simulink model "line_choices_snt"  (R2025b)
settings: Solver=ode45  StartTime=0.0  StopTime=10.0  RelTol=1e-3  EnableMultiTasking=on
values from neighbouring files (symbols this model uses):
  ft2km = 0.0003048    [IEEE_123_data.m]    (also in IEEE_123_data_fault.m)
undefined symbols (not defined in the file or in its folder): C_1, find_system, L_1, R_1
libraries: fl_lib x156, nesl_utility x24
(part 1 of 2)
settings Model: Creator=gdudgeon  LastModifiedBy=gdudgeon
settings SolverCC: AlgebraicLoopSolver=TrustRegion
settings DataIOCC: LimitDataPoints=on  SaveFormat=Array  ReturnWorkspaceOutputs=off
settings OptimizationCC: ExpressionDepthLimit=2147483647.0  LifeSpan=inf
settings DebuggingCC: UnderspecifiedInitializationDetection=Classic  MergeDetectMultiDrivingBlocksExec=none  SolverPrmCheckMsg=warning  UnconnectedInputMsg=warning  UnconnectedOutputMsg=warning  UnconnectedLineMsg=warning  StateNameClashWarn=warning  SFUnexpectedBacktrackingDiag=warning  SFNoUnconditionalDefaultTransitionDiag=warning  SFExecutionAtInitializationDiag=none  ArithmeticOperatorsInVariantConditions=warning
settings HardwareCC: ProdBitPerPointer=32.0  ProdBitPerSizeT=32.0  ProdBitPerPtrDiffT=32.0  ProdLargestAtomicFloat=None  ProdIntDivRoundTo=Undefined  ProdEndianess=Unspecified  ProdWordSize=32.0  ProdHWDeviceType=32-bit Generic
settings ModelReferenceCC: EnableRefExpFcnMdlSchedulingChecks=on  PropagateSignalLabelsOutOfModel=off
settings SFSimCC: SimUseLocalCustomCode=off  CustomCodeUndefinedFunction=UseInterfaceOnly
settings RTWCC: RTWUseLocalCustomCode=off  GPUComputeCapability=3.5
settings CodeAppCC: StateflowObjectComments=on
settings GRTTargetCC: TargetLangStandard=C89/C90 (ANSI)
settings ConfigComp: CovMetricSettings=dw  CovSaveCumulativeToWorkspaceVar=on  CovSaveSingleToWorkspaceVar=on  CovExternalEMLEnable=off  CovSFcnEnable=off
settings SimscapeCC: SimscapeNormalizeSystem=off

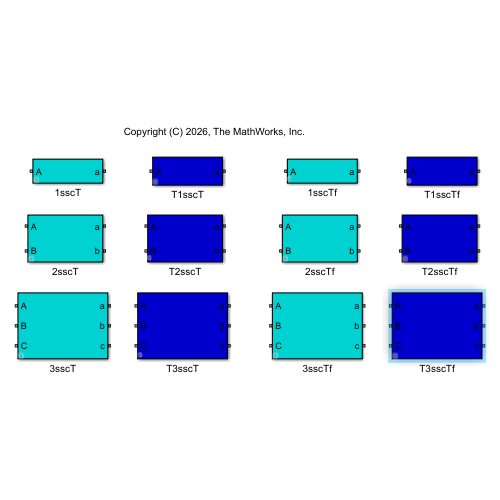
[thumbnail: Simulink's stored preview of the top-level diagram]
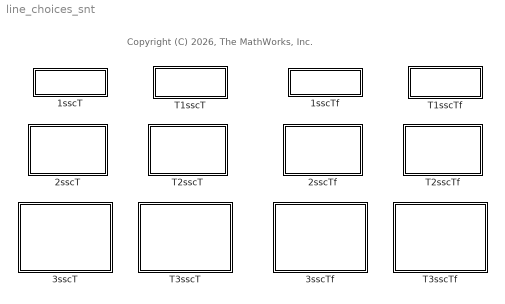
== system line_choices_snt ==
  note: Copyright (C) 2026, The MathWorks, Inc.
  1sscT : Subsystem  mask{from_bus=1, to_bus=7, config=1, length=300}
      mask prompts: from_bus "From Bus"; to_bus "To Bus"; config "Configuration"; length "Length (ft)"
  1sscTf : Subsystem  mask{from_bus=1, to_bus=7, config=1, length=300}
      mask prompts: from_bus "From Bus"; to_bus "To Bus"; config "Configuration"; length "Length (ft)"
  2sscT : Subsystem  mask{from_bus=1, to_bus=7, config=1, length=300}
      mask prompts: from_bus "From Bus"; to_bus "To Bus"; config "Configuration"; length "Length (ft)"
  2sscTf : Subsystem  mask{from_bus=1, to_bus=7, config=1, length=300}
      mask prompts: from_bus "From Bus"; to_bus "To Bus"; config "Configuration"; length "Length (ft)"
  3sscT : Subsystem  mask{from_bus=1, to_bus=7, config=1, length=300}
      mask prompts: from_bus "From Bus"; to_bus "To Bus"; config "Configuration"; length "Length (ft)"
  3sscTf : Subsystem  mask{from_bus=1, to_bus=7, config=1, length=300}
      mask prompts: from_bus "From Bus"; to_bus "To Bus"; config "Configuration"; length "Length (ft)"
  T1sscT : Subsystem  mask{from_bus=67, to_bus=160, config=6, length=350}
      mask prompts: from_bus "From Bus"; to_bus "To Bus"; config "Configuration"; length "Length (ft)"
  T1sscTf : Subsystem  mask{from_bus=67, to_bus=160, config=6, length=350}
      mask prompts: from_bus "From Bus"; to_bus "To Bus"; config "Configuration"; length "Length (ft)"
  T2sscT : Subsystem  mask{from_bus=67, to_bus=160, config=6, length=350}
      mask prompts: from_bus "From Bus"; to_bus "To Bus"; config "Configuration"; length "Length (ft)"
  T2sscTf : Subsystem  mask{from_bus=67, to_bus=160, config=6, length=350}
      mask prompts: from_bus "From Bus"; to_bus "To Bus"; config "Configuration"; length "Length (ft)"
  T3sscT : Subsystem  mask{from_bus=67, to_bus=160, config=6, length=350}
      mask prompts: from_bus "From Bus"; to_bus "To Bus"; config "Configuration"; length "Length (ft)"
  T3sscTf : Subsystem  mask{from_bus=67, to_bus=160, config=6, length=350}
      mask prompts: from_bus "From Bus"; to_bus "To Bus"; config "Configuration"; length "Length (ft)"

== system line_choices_snt/1sscT ==
  Pi-Section Line : Subsystem  mask{Resistance=R_1, Inductance=L_1, Capacitance=C_1, Length=300*ft2km}
      mask prompts: Resistance "R (3x3) ohms/km"; Inductance "L (3x3) H/km"; Capacitance "C (3x3) F/km"; Length "length (km)"
      mask init:
      | R = Resistance*Length;
      | L = Inductance*Length;
      | C = Capacitance*Length;
  A : PMIOPort  Side=Left
  a : PMIOPort  Port=2  Side=Right
  tag scope: Iabc_1=global
  wires:
  Pi-Section Line/1(Imeas) -> [Iabc_1]
  connections:
  a/RConn1 -- Pi-Section Line/RConn1
  A/RConn1 -- Pi-Section Line/LConn1

== system line_choices_snt/1sscTf ==
  Pi-Section Line : Subsystem  mask{Resistance=R_1, Inductance=L_1, Capacitance=C_1, Length=300*ft2km}
      mask prompts: Resistance "R (3x3) ohms/km"; Inductance "L (3x3) H/km"; Capacitance "C (3x3) F/km"; Length "length (km)"
      mask init:
      | R = Resistance*Length;
      | L = Inductance*Length;
      | C = Capacitance*Length;
  A : PMIOPort  Side=Left
  a : PMIOPort  Port=2  Side=Right
  tag scope: Iabc_1=global
  wires:
  Pi-Section Line/1(Imeas) -> [Iabc_1]
  connections:
  A/RConn1 -- Pi-Section Line/LConn1
  a/RConn1 -- Pi-Section Line/RConn1

== system line_choices_snt/2sscT ==
  Pi-Section Line : Subsystem  mask{Resistance=R_1, Inductance=L_1, Capacitance=C_1, Length=300*ft2km}
      mask prompts: Resistance "R (3x3) ohms/km"; Inductance "L (3x3) H/km"; Capacitance "C (3x3) F/km"; Length "length (km)"
      mask init:
      | R = Resistance*Length;
      | L = Inductance*Length;
      | C = Capacitance*Length;
  A : PMIOPort  Side=Left
  a : PMIOPort  Port=2  Side=Right
  B : PMIOPort  Port=3  Side=Left
  b : PMIOPort  Port=4  Side=Right
  tag scope: Iabc_1=global
  wires:
  Pi-Section Line/1(Imeas) -> [Iabc_1]
  connections:
  a/RConn1 -- Pi-Section Line/RConn1
  b/RConn1 -- Pi-Section Line/RConn2
  A/RConn1 -- Pi-Section Line/LConn1
  B/RConn1 -- Pi-Section Line/LConn2

== system line_choices_snt/2sscTf ==
  Pi-Section Line : Subsystem  mask{Resistance=R_1, Inductance=L_1, Capacitance=C_1, Length=300*ft2km}
      mask prompts: Resistance "R (3x3) ohms/km"; Inductance "L (3x3) H/km"; Capacitance "C (3x3) F/km"; Length "length (km)"
      mask init:
      | R = Resistance*Length;
      | L = Inductance*Length;
      | C = Capacitance*Length;
  A : PMIOPort  Side=Left
  a : PMIOPort  Port=2  Side=Right
  B : PMIOPort  Port=3  Side=Left
  b : PMIOPort  Port=4  Side=Right
  tag scope: Iabc_1=global
  wires:
  Pi-Section Line/1(Imeas) -> [Iabc_1]
  connections:
  B/RConn1 -- Pi-Section Line/LConn2
  A/RConn1 -- Pi-Section Line/LConn1
  b/RConn1 -- Pi-Section Line/RConn2
  a/RConn1 -- Pi-Section Line/RConn1

== system line_choices_snt/3sscT ==
  Pi-Section Line : Subsystem  mask{Resistance=R_1, Inductance=L_1, Capacitance=C_1/2, Length=300*ft2km}
      mask prompts: Resistance "R (3x3) ohms/km"; Inductance "L (3x3) H/km"; Capacitance "C (3x3) F/km"; Length "length (km)"
      mask init:
      | R = Resistance*Length;
      | L = Inductance*Length;
      | C = Capacitance*Length;
  A : PMIOPort  Side=Left
  a : PMIOPort  Port=2  Side=Right
  B : PMIOPort  Port=3  Side=Left
  b : PMIOPort  Port=4  Side=Right
  C : PMIOPort  Port=5  Side=Left
  c : PMIOPort  Port=6  Side=Right
  tag scope: Iabc_1=global
  wires:
  Pi-Section Line/1(Imeas) -> [Iabc_1]
  connections:
  c/RConn1 -- Pi-Section Line/RConn3
  b/RConn1 -- Pi-Section Line/RConn2
  a/RConn1 -- Pi-Section Line/RConn1
  C/RConn1 -- Pi-Section Line/LConn3
  B/RConn1 -- Pi-Section Line/LConn2
  A/RConn1 -- Pi-Section Line/LConn1

== system line_choices_snt/3sscTf ==
  Pi-Section Line : Subsystem  mask{Resistance=R_1, Inductance=L_1, Capacitance=C_1/2, Length=300*ft2km}
      mask prompts: Resistance "R (3x3) ohms/km"; Inductance "L (3x3) H/km"; Capacitance "C (3x3) F/km"; Length "length (km)"
      mask init:
      | R = Resistance*Length;
      | L = Inductance*Length;
      | C = Capacitance*Length;
  A : PMIOPort  Side=Left
  a : PMIOPort  Port=2  Side=Right
  B : PMIOPort  Port=3  Side=Left
  b : PMIOPort  Port=4  Side=Right
  C : PMIOPort  Port=5  Side=Left
  c : PMIOPort  Port=6  Side=Right
  tag scope: Iabc_1=global
  wires:
  Pi-Section Line/1(Imeas) -> [Iabc_1]
  connections:
  A/RConn1 -- Pi-Section Line/LConn1
  B/RConn1 -- Pi-Section Line/LConn2
  C/RConn1 -- Pi-Section Line/LConn3
  a/RConn1 -- Pi-Section Line/RConn1
  b/RConn1 -- Pi-Section Line/RConn2
  c/RConn1 -- Pi-Section Line/RConn3

== system line_choices_snt/T1sscT ==
  OLTC : Subsystem  LoadFcn=find_system(gcs,'FollowLinks', 'on', 'LookUnderMasks', 'all');
  Pi-Section Line : Subsystem  mask{Resistance=R_1, Inductance=L_1, Capacitance=C_1, Length=300*ft2km}
      mask prompts: Resistance "R (3x3) ohms/km"; Inductance "L (3x3) H/km"; Capacitance "C (3x3) F/km"; Length "length (km)"
      mask init:
      | R = Resistance*Length;
      | L = Inductance*Length;
      | C = Capacitance*Length;
  A : PMIOPort  Side=Left
  a : PMIOPort  Port=2  Side=Right
  tag scope: Iabc_1=global
  wires:
  Pi-Section Line/1(Imeas) -> [Iabc_1]
  connections:
  A/RConn1 -- OLTC/LConn1
  Pi-Section Line/RConn1 -- a/RConn1
  Pi-Section Line/LConn1 -- OLTC/RConn1

== system line_choices_snt/T1sscTf ==
  OLTC : Subsystem  LoadFcn=find_system(gcs,'FollowLinks', 'on', 'LookUnderMasks', 'all');
  Pi-Section Line : Subsystem  mask{Resistance=R_1, Inductance=L_1, Capacitance=C_1, Length=300*ft2km}
      mask prompts: Resistance "R (3x3) ohms/km"; Inductance "L (3x3) H/km"; Capacitance "C (3x3) F/km"; Length "length (km)"
      mask init:
      | R = Resistance*Length;
      | L = Inductance*Length;
      | C = Capacitance*Length;
  A : PMIOPort  Side=Left
  a : PMIOPort  Port=2  Side=Right
  tag scope: Iabc_1=global
  wires:
  Pi-Section Line/1(Imeas) -> [Iabc_1]
  connections:
  Pi-Section Line/LConn1 -- OLTC/RConn1
  Pi-Section Line/RConn1 -- a/RConn1
  A/RConn1 -- OLTC/LConn1

== system line_choices_snt/T2sscT ==
  OLTC : Subsystem  LoadFcn=find_system(gcs,'FollowLinks', 'on', 'LookUnderMasks', 'all');
  Pi-Section Line : Subsystem  mask{Resistance=R_1, Inductance=L_1, Capacitance=C_1, Length=300*ft2km}
      mask prompts: Resistance "R (3x3) ohms/km"; Inductance "L (3x3) H/km"; Capacitance "C (3x3) F/km"; Length "length (km)"
      mask init:
      | R = Resistance*Length;
      | L = Inductance*Length;
      | C = Capacitance*Length;
  A : PMIOPort  Side=Left
  a : PMIOPort  Port=2  Side=Right
  B : PMIOPort  Port=3  Side=Left
  b : PMIOPort  Port=4  Side=Right
  tag scope: Iabc_1=global
  wires:
  Pi-Section Line/1(Imeas) -> [Iabc_1]
  connections:
  a/RConn1 -- Pi-Section Line/RConn1
  b/RConn1 -- Pi-Section Line/RConn2
  A/RConn1 -- OLTC/LConn1
  B/RConn1 -- OLTC/LConn2
  Pi-Section Line/LConn2 -- OLTC/RConn2
  Pi-Section Line/LConn1 -- OLTC/RConn1

== system line_choices_snt/T2sscTf ==
  OLTC : Subsystem  LoadFcn=find_system(gcs,'FollowLinks', 'on', 'LookUnderMasks', 'all');
  Pi-Section Line : Subsystem  mask{Resistance=R_1, Inductance=L_1, Capacitance=C_1, Length=300*ft2km}
      mask prompts: Resistance "R (3x3) ohms/km"; Inductance "L (3x3) H/km"; Capacitance "C (3x3) F/km"; Length "length (km)"
      mask init:
      | R = Resistance*Length;
      | L = Inductance*Length;
      | C = Capacitance*Length;
  A : PMIOPort  Side=Left
  a : PMIOPort  Port=2  Side=Right
  B : PMIOPort  Port=3  Side=Left
  b : PMIOPort  Port=4  Side=Right
  tag scope: Iabc_1=global
  wires:
  Pi-Section Line/1(Imeas) -> [Iabc_1]
  connections:
  Pi-Section Line/LConn1 -- OLTC/RConn1
  Pi-Section Line/LConn2 -- OLTC/RConn2
  B/RConn1 -- OLTC/LConn2
  A/RConn1 -- OLTC/LConn1
  b/RConn1 -- Pi-Section Line/RConn2
  a/RConn1 -- Pi-Section Line/RConn1

== system line_choices_snt/T3sscT ==
  OLTC : Subsystem  LoadFcn=find_system(gcs,'FollowLinks', 'on', 'LookUnderMasks', 'all');
  Pi-Section Line : Subsystem  mask{Resistance=R_1, Inductance=L_1, Capacitance=C_1/2, Length=300*ft2km}
      mask prompts: Resistance "R (3x3) ohms/km"; Inductance "L (3x3) H/km"; Capacitance "C (3x3) F/km"; Length "length (km)"
      mask init:
      | R = Resistance*Length;
      | L = Inductance*Length;
      | C = Capacitance*Length;
  A : PMIOPort  Side=Left
  a : PMIOPort  Port=2  Side=Right
  B : PMIOPort  Port=3  Side=Left
  b : PMIOPort  Port=4  Side=Right
  C : PMIOPort  Port=5  Side=Left
  c : PMIOPort  Port=6  Side=Right
  tag scope: Iabc_1=global
  wires:
  Pi-Section Line/1(Imeas) -> [Iabc_1]
  connections:
  A/RConn1 -- OLTC/LConn1
  B/RConn1 -- OLTC/LConn2
  OLTC/LConn3 -- C/RConn1
  c/RConn1 -- Pi-Section Line/RConn3
  Pi-Section Line/RConn1 -- a/RConn1
  b/RConn1 -- Pi-Section Line/RConn2
  Pi-Section Line/LConn2 -- OLTC/RConn2
  OLTC/RConn1 -- Pi-Section Line/LConn1
  OLTC/RConn3 -- Pi-Section Line/LConn3

== system line_choices_snt/T3sscTf ==
  OLTC : Subsystem  LoadFcn=find_system(gcs,'FollowLinks', 'on', 'LookUnderMasks', 'all');
  Pi-Section Line : Subsystem  mask{Resistance=R_1, Inductance=L_1, Capacitance=C_1/2, Length=300*ft2km}
      mask prompts: Resistance "R (3x3) ohms/km"; Inductance "L (3x3) H/km"; Capacitance "C (3x3) F/km"; Length "length (km)"
      mask init:
      | R = Resistance*Length;
      | L = Inductance*Length;
      | C = Capacitance*Length;
  A : PMIOPort  Side=Left
  a : PMIOPort  Port=2  Side=Right
  B : PMIOPort  Port=3  Side=Left
  b : PMIOPort  Port=4  Side=Right
  C : PMIOPort  Port=5  Side=Left
  c : PMIOPort  Port=6  Side=Right
  tag scope: Iabc_1=global
  wires:
  Pi-Section Line/1(Imeas) -> [Iabc_1]
  connections:
  OLTC/RConn3 -- Pi-Section Line/LConn3
  OLTC/RConn1 -- Pi-Section Line/LConn1
  Pi-Section Line/LConn2 -- OLTC/RConn2
  b/RConn1 -- Pi-Section Line/RConn2
  Pi-Section Line/RConn1 -- a/RConn1
  c/RConn1 -- Pi-Section Line/RConn3
  OLTC/LConn3 -- C/RConn1
  B/RConn1 -- OLTC/LConn2
  A/RConn1 -- OLTC/LConn1

== system line_choices_snt/1sscT/Pi-Section Line ==
  Electrical Reference : fl_lib/Electrical/Electrical Elements/Electrical Reference
  Electrical Reference1 : fl_lib/Electrical/Electrical Elements/Electrical Reference
  Mutual C1 : SimscapeComponentBlock  SourceFile=multi_coupled_C  ComponentPath=multi_coupled_C  ComponentVariants="[\"multi_coupled_C\"]"  ComponentVariantNames="[\"multi_coupled_C\"]"  ClassName=multi_coupled_C  SchemaVersion=1  noph=1  C=C F
      settings: CopyFcn=simscape.sscblock.internal.componentBlockCallback(gcbh,'COPY')  PreCopyFcn=simscape.sscblock.internal.componentBlockCallback(gcbh,'PRECOPY')  PreDeleteFcn=simscape.sscblock.internal.componentBlockCallback(gcbh,'PREDELETE')  InternalSimscapePortConfiguration="{\"Bottom\":[],\"Left\":[{\"id\":\"p\",\"label\":\"p\",\"type\":\"foundation.electrical.electrical\"}],\"Right\":[{\"id\":\"n\",\"label\":\"n\",\"type\":\"foundation.electrical.electrical\"}],\"Top\":[]}"
      mask Type: Multi-Phase Coupled C
  Mutual C2 : SimscapeComponentBlock  SourceFile=multi_coupled_C  ComponentPath=multi_coupled_C  ComponentVariants="[\"multi_coupled_C\"]"  ComponentVariantNames="[\"multi_coupled_C\"]"  ClassName=multi_coupled_C  SchemaVersion=1  noph=1  C=C F
      settings: CopyFcn=simscape.sscblock.internal.componentBlockCallback(gcbh,'COPY')  PreCopyFcn=simscape.sscblock.internal.componentBlockCallback(gcbh,'PRECOPY')  PreDeleteFcn=simscape.sscblock.internal.componentBlockCallback(gcbh,'PREDELETE')  InternalSimscapePortConfiguration="{\"Bottom\":[],\"Left\":[{\"id\":\"p\",\"label\":\"p\",\"type\":\"foundation.electrical.electrical\"}],\"Right\":[{\"id\":\"n\",\"label\":\"n\",\"type\":\"foundation.electrical.electrical\"}],\"Top\":[]}"
      mask Type: Multi-Phase Coupled C
  Mutual RL : SimscapeComponentBlock  SourceFile=multi_coupled_RL  ComponentPath=multi_coupled_RL  ComponentVariants="[\"multi_coupled_RL\"]"  ComponentVariantNames="[\"multi_coupled_RL\"]"  ClassName=multi_coupled_RL  SchemaVersion=1  noph=1  R=R Ohm  L=L H
      settings: CopyFcn=simscape.sscblock.internal.componentBlockCallback(gcbh,'COPY')  PreCopyFcn=simscape.sscblock.internal.componentBlockCallback(gcbh,'PRECOPY')  PreDeleteFcn=simscape.sscblock.internal.componentBlockCallback(gcbh,'PREDELETE')  InternalSimscapePortConfiguration="{\"Bottom\":[],\"Left\":[{\"id\":\"p\",\"label\":\"p\",\"type\":\"foundation.electrical.electrical\"}],\"Right\":[{\"id\":\"n\",\"label\":\"n\",\"type\":\"foundation.electrical.electrical\"}],\"Top\":[]}"
      mask Type: Multi-Phase Coupled RL
  PS-Simulink Converter : nesl_utility/PS-Simulink Converter  PhysicalDomain=network_engine_domain  SubClassName=ps_output  LeftPortType=input  RightPortType=output  PseudoPeriodic=off  Frequencies=[]  VectorFormat=inherit  Unit=inherit  AffineConversion=off
  Simscape Component : SimscapeComponentBlock  SourceFile=multi_current  ComponentPath=multi_current  ComponentVariants="[\"multi_current\"]"  ComponentVariantNames="[\"multi_current\"]"  ClassName=multi_current  SchemaVersion=1  noph=1
      settings: CopyFcn=simscape.sscblock.internal.componentBlockCallback(gcbh,'COPY')  PreCopyFcn=simscape.sscblock.internal.componentBlockCallback(gcbh,'PRECOPY')  PreDeleteFcn=simscape.sscblock.internal.componentBlockCallback(gcbh,'PREDELETE')  InternalSimscapePortConfiguration="{\"Bottom\":[],\"Left\":[{\"id\":\"p\",\"label\":\"+\",\"type\":\"foundation.electrical.electrical\"}],\"Right\":[{\"id\":\"I\",\"label\":\"I\",\"type\":\"output\"},{\"id\":\"n\",\"label\":\"-\",\"type\":\"foundation.electrical.electrical\"}],\"Top\":[]}"
      mask Type: Multi-Phase Current Sensor
  A : PMIOPort  Side=Left
  a : PMIOPort  Port=2  Side=Right
  Imeas : Outport
  wires:
  PS-Simulink Converter/1 -> Imeas/1
  connections:
  Mutual RL/LConn1 -- Simscape Component/RConn2 -- Mutual C1/LConn1
  Mutual RL/RConn1 -- a/RConn1 -- Mutual C2/LConn1
  Mutual C1/RConn1 -- Electrical Reference/LConn1
  Mutual C2/RConn1 -- Electrical Reference1/LConn1
  Simscape Component/LConn1 -- A/RConn1
  PS-Simulink Converter/LConn1 -- Simscape Component/RConn1

== system line_choices_snt/1sscTf/Pi-Section Line ==
  Electrical Reference : fl_lib/Electrical/Electrical Elements/Electrical Reference
  Electrical Reference1 : fl_lib/Electrical/Electrical Elements/Electrical Reference
  Mutual C1 : SimscapeComponentBlock  SourceFile=multi_coupled_C  ComponentPath=multi_coupled_C  ComponentVariants="[\"multi_coupled_C\"]"  ComponentVariantNames="[\"multi_coupled_C\"]"  ClassName=multi_coupled_C  SchemaVersion=1  noph=1  C=C F
      settings: CopyFcn=simscape.sscblock.internal.componentBlockCallback(gcbh,'COPY')  PreCopyFcn=simscape.sscblock.internal.componentBlockCallback(gcbh,'PRECOPY')  PreDeleteFcn=simscape.sscblock.internal.componentBlockCallback(gcbh,'PREDELETE')  InternalSimscapePortConfiguration="{\"Bottom\":[],\"Left\":[{\"id\":\"p\",\"label\":\"p\",\"type\":\"foundation.electrical.electrical\"}],\"Right\":[{\"id\":\"n\",\"label\":\"n\",\"type\":\"foundation.electrical.electrical\"}],\"Top\":[]}"
      mask Type: Multi-Phase Coupled C
  Mutual C2 : SimscapeComponentBlock  SourceFile=multi_coupled_C  ComponentPath=multi_coupled_C  ComponentVariants="[\"multi_coupled_C\"]"  ComponentVariantNames="[\"multi_coupled_C\"]"  ClassName=multi_coupled_C  SchemaVersion=1  noph=1  C=C F
      settings: CopyFcn=simscape.sscblock.internal.componentBlockCallback(gcbh,'COPY')  PreCopyFcn=simscape.sscblock.internal.componentBlockCallback(gcbh,'PRECOPY')  PreDeleteFcn=simscape.sscblock.internal.componentBlockCallback(gcbh,'PREDELETE')  InternalSimscapePortConfiguration="{\"Bottom\":[],\"Left\":[{\"id\":\"p\",\"label\":\"p\",\"type\":\"foundation.electrical.electrical\"}],\"Right\":[{\"id\":\"n\",\"label\":\"n\",\"type\":\"foundation.electrical.electrical\"}],\"Top\":[]}"
      mask Type: Multi-Phase Coupled C
  Mutual RL : SimscapeComponentBlock  SourceFile=multi_coupled_RL  ComponentPath=multi_coupled_RL  ComponentVariants="[\"multi_coupled_RL\"]"  ComponentVariantNames="[\"multi_coupled_RL\"]"  ClassName=multi_coupled_RL  SchemaVersion=1  noph=1  R=R Ohm  L=L H
      settings: CopyFcn=simscape.sscblock.internal.componentBlockCallback(gcbh,'COPY')  PreCopyFcn=simscape.sscblock.internal.componentBlockCallback(gcbh,'PRECOPY')  PreDeleteFcn=simscape.sscblock.internal.componentBlockCallback(gcbh,'PREDELETE')  InternalSimscapePortConfiguration="{\"Bottom\":[],\"Left\":[{\"id\":\"p\",\"label\":\"p\",\"type\":\"foundation.electrical.electrical\"}],\"Right\":[{\"id\":\"n\",\"label\":\"n\",\"type\":\"foundation.electrical.electrical\"}],\"Top\":[]}"
      mask Type: Multi-Phase Coupled RL
  PS-Simulink Converter : nesl_utility/PS-Simulink Converter  PhysicalDomain=network_engine_domain  SubClassName=ps_output  LeftPortType=input  RightPortType=output  PseudoPeriodic=off  Frequencies=[]  VectorFormat=inherit  Unit=inherit  AffineConversion=off
  Simscape Component : SimscapeComponentBlock  SourceFile=multi_current  ComponentPath=multi_current  ComponentVariants="[\"multi_current\"]"  ComponentVariantNames="[\"multi_current\"]"  ClassName=multi_current  SchemaVersion=1  noph=1
      settings: CopyFcn=simscape.sscblock.internal.componentBlockCallback(gcbh,'COPY')  PreCopyFcn=simscape.sscblock.internal.componentBlockCallback(gcbh,'PRECOPY')  PreDeleteFcn=simscape.sscblock.internal.componentBlockCallback(gcbh,'PREDELETE')  InternalSimscapePortConfiguration="{\"Bottom\":[],\"Left\":[{\"id\":\"p\",\"label\":\"+\",\"type\":\"foundation.electrical.electrical\"}],\"Right\":[{\"id\":\"I\",\"label\":\"I\",\"type\":\"output\"},{\"id\":\"n\",\"label\":\"-\",\"type\":\"foundation.electrical.electrical\"}],\"Top\":[]}"
      mask Type: Multi-Phase Current Sensor
  A : PMIOPort  Side=Left
  a : PMIOPort  Port=2  Side=Right
  Imeas : Outport
  wires:
  PS-Simulink Converter/1 -> Imeas/1
  connections:
  PS-Simulink Converter/LConn1 -- Simscape Component/RConn1
  Simscape Component/LConn1 -- A/RConn1
  Mutual C2/RConn1 -- Electrical Reference1/LConn1
  Mutual C1/RConn1 -- Electrical Reference/LConn1
  Mutual C2/LConn1 -- a/RConn1 -- Mutual RL/RConn1
  Mutual C1/LConn1 -- Simscape Component/RConn2 -- Mutual RL/LConn1

== system line_choices_snt/2sscT/Pi-Section Line ==
  Array Connection{,1..3} (4 alike) : SimscapeArrayConnection
  Electrical Reference : fl_lib/Electrical/Electrical Elements/Electrical Reference
  Electrical Reference1 : fl_lib/Electrical/Electrical Elements/Electrical Reference
  Mutual C1 : SimscapeComponentBlock  SourceFile=multi_coupled_C  ComponentPath=multi_coupled_C  ComponentVariants="[\"multi_coupled_C\"]"  ComponentVariantNames="[\"multi_coupled_C\"]"  ClassName=multi_coupled_C  SchemaVersion=1  noph=2  C=C F
      settings: CopyFcn=simscape.sscblock.internal.componentBlockCallback(gcbh,'COPY')  PreCopyFcn=simscape.sscblock.internal.componentBlockCallback(gcbh,'PRECOPY')  PreDeleteFcn=simscape.sscblock.internal.componentBlockCallback(gcbh,'PREDELETE')  InternalSimscapePortConfiguration="{\"Bottom\":[],\"Left\":[{\"id\":\"p\",\"label\":\"p\",\"type\":\"foundation.electrical.electrical\"}],\"Right\":[{\"id\":\"n\",\"label\":\"n\",\"type\":\"foundation.electrical.electrical\"}],\"Top\":[]}"
      mask Type: Multi-Phase Coupled C
  Mutual C2 : SimscapeComponentBlock  SourceFile=multi_coupled_C  ComponentPath=multi_coupled_C  ComponentVariants="[\"multi_coupled_C\"]"  ComponentVariantNames="[\"multi_coupled_C\"]"  ClassName=multi_coupled_C  SchemaVersion=1  noph=2  C=C F
      settings: CopyFcn=simscape.sscblock.internal.componentBlockCallback(gcbh,'COPY')  PreCopyFcn=simscape.sscblock.internal.componentBlockCallback(gcbh,'PRECOPY')  PreDeleteFcn=simscape.sscblock.internal.componentBlockCallback(gcbh,'PREDELETE')  InternalSimscapePortConfiguration="{\"Bottom\":[],\"Left\":[{\"id\":\"p\",\"label\":\"p\",\"type\":\"foundation.electrical.electrical\"}],\"Right\":[{\"id\":\"n\",\"label\":\"n\",\"type\":\"foundation.electrical.electrical\"}],\"Top\":[]}"
      mask Type: Multi-Phase Coupled C
  Mutual RL : SimscapeComponentBlock  SourceFile=multi_coupled_RL  ComponentPath=multi_coupled_RL  ComponentVariants="[\"multi_coupled_RL\"]"  ComponentVariantNames="[\"multi_coupled_RL\"]"  ClassName=multi_coupled_RL  SchemaVersion=1  noph=2  R=R Ohm  L=L H
      settings: CopyFcn=simscape.sscblock.internal.componentBlockCallback(gcbh,'COPY')  PreCopyFcn=simscape.sscblock.internal.componentBlockCallback(gcbh,'PRECOPY')  PreDeleteFcn=simscape.sscblock.internal.componentBlockCallback(gcbh,'PREDELETE')  InternalSimscapePortConfiguration="{\"Bottom\":[],\"Left\":[{\"id\":\"p\",\"label\":\"p\",\"type\":\"foundation.electrical.electrical\"}],\"Right\":[{\"id\":\"n\",\"label\":\"n\",\"type\":\"foundation.electrical.electrical\"}],\"Top\":[]}"
      mask Type: Multi-Phase Coupled RL
  PS-Simulink Converter : nesl_utility/PS-Simulink Converter  PhysicalDomain=network_engine_domain  SubClassName=ps_output  LeftPortType=input  RightPortType=output  PseudoPeriodic=off  Frequencies=[]  VectorFormat=inherit  Unit=inherit  AffineConversion=off
  Simscape Component : SimscapeComponentBlock  SourceFile=multi_current  ComponentPath=multi_current  ComponentVariants="[\"multi_current\"]"  ComponentVariantNames="[\"multi_current\"]"  ClassName=multi_current  SchemaVersion=1  noph=2
      settings: CopyFcn=simscape.sscblock.internal.componentBlockCallback(gcbh,'COPY')  PreCopyFcn=simscape.sscblock.internal.componentBlockCallback(gcbh,'PRECOPY')  PreDeleteFcn=simscape.sscblock.internal.componentBlockCallback(gcbh,'PREDELETE')  InternalSimscapePortConfiguration="{\"Bottom\":[],\"Left\":[{\"id\":\"p\",\"label\":\"+\",\"type\":\"foundation.electrical.electrical\"}],\"Right\":[{\"id\":\"I\",\"label\":\"I\",\"type\":\"output\"},{\"id\":\"n\",\"label\":\"-\",\"type\":\"foundation.electrical.electrical\"}],\"Top\":[]}"
      mask Type: Multi-Phase Current Sensor
  A : PMIOPort  Side=Left
  B : PMIOPort  Port=2  Side=Left
  a : PMIOPort  Port=3  Side=Right
  b : PMIOPort  Port=4  Side=Right
  Imeas : Outport
  wires:
  PS-Simulink Converter/1 -> Imeas/1
  connections:
  Mutual RL/RConn1 -- Array Connection1/RConn1 -- Mutual C2/LConn1
  Mutual C1/LConn1 -- Simscape Component/RConn2 -- Mutual RL/LConn1
  PS-Simulink Converter/LConn1 -- Simscape Component/RConn1
  Array Connection/RConn1 -- Simscape Component/LConn1
  A/RConn1 -- Array Connection/LConn1
  B/RConn1 -- Array Connection/LConn2
  a/RConn1 -- Array Connection1/LConn1
  b/RConn1 -- Array Connection1/LConn2
  Array Connection2/RConn1 -- Mutual C1/RConn1
  Array Connection3/RConn1 -- Mutual C2/RConn1
  Array Connection2/LConn1 -- Electrical Reference/LConn1 -- Array Connection2/LConn2
  Array Connection3/LConn1 -- Electrical Reference1/LConn1 -- Array Connection3/LConn2

== system line_choices_snt/2sscTf/Pi-Section Line ==
  Array Connection{,1..3} (4 alike) : SimscapeArrayConnection
  Electrical Reference : fl_lib/Electrical/Electrical Elements/Electrical Reference
  Electrical Reference1 : fl_lib/Electrical/Electrical Elements/Electrical Reference
  Mutual C1 : SimscapeComponentBlock  SourceFile=multi_coupled_C  ComponentPath=multi_coupled_C  ComponentVariants="[\"multi_coupled_C\"]"  ComponentVariantNames="[\"multi_coupled_C\"]"  ClassName=multi_coupled_C  SchemaVersion=1  noph=2  C=C F
      settings: CopyFcn=simscape.sscblock.internal.componentBlockCallback(gcbh,'COPY')  PreCopyFcn=simscape.sscblock.internal.componentBlockCallback(gcbh,'PRECOPY')  PreDeleteFcn=simscape.sscblock.internal.componentBlockCallback(gcbh,'PREDELETE')  InternalSimscapePortConfiguration="{\"Bottom\":[],\"Left\":[{\"id\":\"p\",\"label\":\"p\",\"type\":\"foundation.electrical.electrical\"}],\"Right\":[{\"id\":\"n\",\"label\":\"n\",\"type\":\"foundation.electrical.electrical\"}],\"Top\":[]}"
      mask Type: Multi-Phase Coupled C
  Mutual C2 : SimscapeComponentBlock  SourceFile=multi_coupled_C  ComponentPath=multi_coupled_C  ComponentVariants="[\"multi_coupled_C\"]"  ComponentVariantNames="[\"multi_coupled_C\"]"  ClassName=multi_coupled_C  SchemaVersion=1  noph=2  C=C F
      settings: CopyFcn=simscape.sscblock.internal.componentBlockCallback(gcbh,'COPY')  PreCopyFcn=simscape.sscblock.internal.componentBlockCallback(gcbh,'PRECOPY')  PreDeleteFcn=simscape.sscblock.internal.componentBlockCallback(gcbh,'PREDELETE')  InternalSimscapePortConfiguration="{\"Bottom\":[],\"Left\":[{\"id\":\"p\",\"label\":\"p\",\"type\":\"foundation.electrical.electrical\"}],\"Right\":[{\"id\":\"n\",\"label\":\"n\",\"type\":\"foundation.electrical.electrical\"}],\"Top\":[]}"
      mask Type: Multi-Phase Coupled C
  Mutual RL : SimscapeComponentBlock  SourceFile=multi_coupled_RL  ComponentPath=multi_coupled_RL  ComponentVariants="[\"multi_coupled_RL\"]"  ComponentVariantNames="[\"multi_coupled_RL\"]"  ClassName=multi_coupled_RL  SchemaVersion=1  noph=2  R=R Ohm  L=L H
      settings: CopyFcn=simscape.sscblock.internal.componentBlockCallback(gcbh,'COPY')  PreCopyFcn=simscape.sscblock.internal.componentBlockCallback(gcbh,'PRECOPY')  PreDeleteFcn=simscape.sscblock.internal.componentBlockCallback(gcbh,'PREDELETE')  InternalSimscapePortConfiguration="{\"Bottom\":[],\"Left\":[{\"id\":\"p\",\"label\":\"p\",\"type\":\"foundation.electrical.electrical\"}],\"Right\":[{\"id\":\"n\",\"label\":\"n\",\"type\":\"foundation.electrical.electrical\"}],\"Top\":[]}"
      mask Type: Multi-Phase Coupled RL
  PS-Simulink Converter : nesl_utility/PS-Simulink Converter  PhysicalDomain=network_engine_domain  SubClassName=ps_output  LeftPortType=input  RightPortType=output  PseudoPeriodic=off  Frequencies=[]  VectorFormat=inherit  Unit=inherit  AffineConversion=off
  Simscape Component : SimscapeComponentBlock  SourceFile=multi_current  ComponentPath=multi_current  ComponentVariants="[\"multi_current\"]"  ComponentVariantNames="[\"multi_current\"]"  ClassName=multi_current  SchemaVersion=1  noph=2
      settings: CopyFcn=simscape.sscblock.internal.componentBlockCallback(gcbh,'COPY')  PreCopyFcn=simscape.sscblock.internal.componentBlockCallback(gcbh,'PRECOPY')  PreDeleteFcn=simscape.sscblock.internal.componentBlockCallback(gcbh,'PREDELETE')  InternalSimscapePortConfiguration="{\"Bottom\":[],\"Left\":[{\"id\":\"p\",\"label\":\"+\",\"type\":\"foundation.electrical.electrical\"}],\"Right\":[{\"id\":\"I\",\"label\":\"I\",\"type\":\"output\"},{\"id\":\"n\",\"label\":\"-\",\"type\":\"foundation.electrical.electrical\"}],\"Top\":[]}"
      mask Type: Multi-Phase Current Sensor
  A : PMIOPort  Side=Left
  B : PMIOPort  Port=2  Side=Left
  a : PMIOPort  Port=3  Side=Right
  b : PMIOPort  Port=4  Side=Right
  Imeas : Outport
  wires:
  PS-Simulink Converter/1 -> Imeas/1
  connections:
  Array Connection3/LConn2 -- Electrical Reference1/LConn1 -- Array Connection3/LConn1
  Array Connection2/LConn2 -- Electrical Reference/LConn1 -- Array Connection2/LConn1
  Array Connection3/RConn1 -- Mutual C2/RConn1
  Array Connection2/RConn1 -- Mutual C1/RConn1
  b/RConn1 -- Array Connection1/LConn2
  a/RConn1 -- Array Connection1/LConn1
  B/RConn1 -- Array Connection/LConn2
  A/RConn1 -- Array Connection/LConn1
  Array Connection/RConn1 -- Simscape Component/LConn1
  PS-Simulink Converter/LConn1 -- Simscape Component/RConn1
  Mutual RL/LConn1 -- Simscape Component/RConn2 -- Mutual C1/LConn1
  Mutual C2/LConn1 -- Array Connection1/RConn1 -- Mutual RL/RConn1

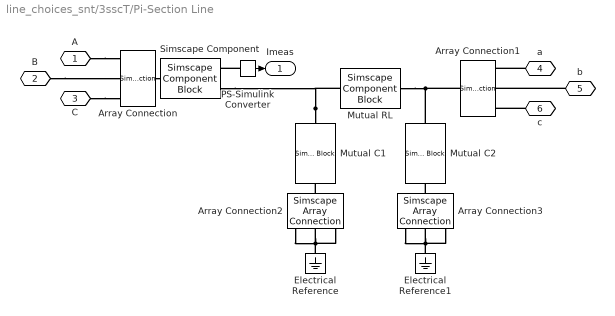
== system line_choices_snt/3sscT/Pi-Section Line ==
  Array Connection{,1..3} (4 alike) : SimscapeArrayConnection  NumScalarElements=3
  Electrical Reference : fl_lib/Electrical/Electrical Elements/Electrical Reference
  Electrical Reference1 : fl_lib/Electrical/Electrical Elements/Electrical Reference
  Mutual C1 : SimscapeComponentBlock  SourceFile=multi_coupled_C  ComponentPath=multi_coupled_C  ComponentVariants="[\"multi_coupled_C\"]"  ComponentVariantNames="[\"multi_coupled_C\"]"  ClassName=multi_coupled_C  SchemaVersion=1  noph=3  C=C F
      settings: CopyFcn=simscape.sscblock.internal.componentBlockCallback(gcbh,'COPY')  PreCopyFcn=simscape.sscblock.internal.componentBlockCallback(gcbh,'PRECOPY')  PreDeleteFcn=simscape.sscblock.internal.componentBlockCallback(gcbh,'PREDELETE')  InternalSimscapePortConfiguration="{\"Bottom\":[],\"Left\":[{\"id\":\"p\",\"label\":\"p\",\"type\":\"foundation.electrical.electrical\"}],\"Right\":[{\"id\":\"n\",\"label\":\"n\",\"type\":\"foundation.electrical.electrical\"}],\"Top\":[]}"
      mask Type: Multi-Phase Coupled C
  Mutual C2 : SimscapeComponentBlock  SourceFile=multi_coupled_C  ComponentPath=multi_coupled_C  ComponentVariants="[\"multi_coupled_C\"]"  ComponentVariantNames="[\"multi_coupled_C\"]"  ClassName=multi_coupled_C  SchemaVersion=1  noph=3  C=C F
      settings: CopyFcn=simscape.sscblock.internal.componentBlockCallback(gcbh,'COPY')  PreCopyFcn=simscape.sscblock.internal.componentBlockCallback(gcbh,'PRECOPY')  PreDeleteFcn=simscape.sscblock.internal.componentBlockCallback(gcbh,'PREDELETE')  InternalSimscapePortConfiguration="{\"Bottom\":[],\"Left\":[{\"id\":\"p\",\"label\":\"p\",\"type\":\"foundation.electrical.electrical\"}],\"Right\":[{\"id\":\"n\",\"label\":\"n\",\"type\":\"foundation.electrical.electrical\"}],\"Top\":[]}"
      mask Type: Multi-Phase Coupled C
  Mutual RL : SimscapeComponentBlock  SourceFile=multi_coupled_RL  ComponentPath=multi_coupled_RL  ComponentVariants="[\"multi_coupled_RL\"]"  ComponentVariantNames="[\"multi_coupled_RL\"]"  ClassName=multi_coupled_RL  SchemaVersion=1  noph=3  R=R Ohm  L=L H
      settings: CopyFcn=simscape.sscblock.internal.componentBlockCallback(gcbh,'COPY')  PreCopyFcn=simscape.sscblock.internal.componentBlockCallback(gcbh,'PRECOPY')  PreDeleteFcn=simscape.sscblock.internal.componentBlockCallback(gcbh,'PREDELETE')  InternalSimscapePortConfiguration="{\"Bottom\":[],\"Left\":[{\"id\":\"p\",\"label\":\"p\",\"type\":\"foundation.electrical.electrical\"}],\"Right\":[{\"id\":\"n\",\"label\":\"n\",\"type\":\"foundation.electrical.electrical\"}],\"Top\":[]}"
      mask Type: Multi-Phase Coupled RL
  PS-Simulink Converter : nesl_utility/PS-Simulink Converter  PhysicalDomain=network_engine_domain  SubClassName=ps_output  LeftPortType=input  RightPortType=output  PseudoPeriodic=off  Frequencies=[]  VectorFormat=inherit  Unit=inherit  AffineConversion=off
  Simscape Component : SimscapeComponentBlock  SourceFile=multi_current  ComponentPath=multi_current  ComponentVariants="[\"multi_current\"]"  ComponentVariantNames="[\"multi_current\"]"  ClassName=multi_current  SchemaVersion=1  noph=3
      settings: CopyFcn=simscape.sscblock.internal.componentBlockCallback(gcbh,'COPY')  PreCopyFcn=simscape.sscblock.internal.componentBlockCallback(gcbh,'PRECOPY')  PreDeleteFcn=simscape.sscblock.internal.componentBlockCallback(gcbh,'PREDELETE')  InternalSimscapePortConfiguration="{\"Bottom\":[],\"Left\":[{\"id\":\"p\",\"label\":\"+\",\"type\":\"foundation.electrical.electrical\"}],\"Right\":[{\"id\":\"I\",\"label\":\"I\",\"type\":\"output\"},{\"id\":\"n\",\"label\":\"-\",\"type\":\"foundation.electrical.electrical\"}],\"Top\":[]}"
      mask Type: Multi-Phase Current Sensor
  A : PMIOPort  Side=Left
  B : PMIOPort  Port=2  Side=Left
  C : PMIOPort  Port=3  Side=Left
  a : PMIOPort  Port=4  Side=Right
  b : PMIOPort  Port=5  Side=Right
  c : PMIOPort  Port=6  Side=Right
  Imeas : Outport
  wires:
  PS-Simulink Converter/1 -> Imeas/1
  connections:
  Array Connection2/LConn2 -- Array Connection2/LConn3 -- Array Connection2/LConn1 -- Electrical Reference/LConn1
  Mutual RL/RConn1 -- Array Connection1/RConn1 -- Mutual C2/LConn1
  Mutual C1/LConn1 -- Simscape Component/RConn2 -- Mutual RL/LConn1
  Array Connection3/LConn1 -- Array Connection3/LConn2 -- Array Connection3/LConn3 -- Electrical Reference1/LConn1
  Array Connection2/RConn1 -- Mutual C1/RConn1
  Array Connection/RConn1 -- Simscape Component/LConn1
  PS-Simulink Converter/LConn1 -- Simscape Component/RConn1
  Array Connection3/RConn1 -- Mutual C2/RConn1
  A/RConn1 -- Array Connection/LConn1
  B/RConn1 -- Array Connection/LConn2
  C/RConn1 -- Array Connection/LConn3
  a/RConn1 -- Array Connection1/LConn1
  b/RConn1 -- Array Connection1/LConn2
  c/RConn1 -- Array Connection1/LConn3

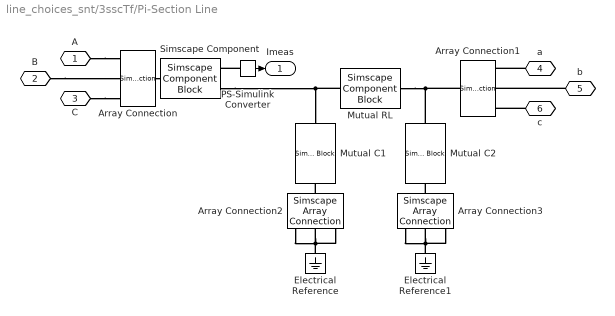
== system line_choices_snt/3sscTf/Pi-Section Line ==
  Array Connection{,1..3} (4 alike) : SimscapeArrayConnection  NumScalarElements=3
  Electrical Reference : fl_lib/Electrical/Electrical Elements/Electrical Reference
  Electrical Reference1 : fl_lib/Electrical/Electrical Elements/Electrical Reference
  Mutual C1 : SimscapeComponentBlock  SourceFile=multi_coupled_C  ComponentPath=multi_coupled_C  ComponentVariants="[\"multi_coupled_C\"]"  ComponentVariantNames="[\"multi_coupled_C\"]"  ClassName=multi_coupled_C  SchemaVersion=1  noph=3  C=C F
      settings: CopyFcn=simscape.sscblock.internal.componentBlockCallback(gcbh,'COPY')  PreCopyFcn=simscape.sscblock.internal.componentBlockCallback(gcbh,'PRECOPY')  PreDeleteFcn=simscape.sscblock.internal.componentBlockCallback(gcbh,'PREDELETE')  InternalSimscapePortConfiguration="{\"Bottom\":[],\"Left\":[{\"id\":\"p\",\"label\":\"p\",\"type\":\"foundation.electrical.electrical\"}],\"Right\":[{\"id\":\"n\",\"label\":\"n\",\"type\":\"foundation.electrical.electrical\"}],\"Top\":[]}"
      mask Type: Multi-Phase Coupled C
  Mutual C2 : SimscapeComponentBlock  SourceFile=multi_coupled_C  ComponentPath=multi_coupled_C  ComponentVariants="[\"multi_coupled_C\"]"  ComponentVariantNames="[\"multi_coupled_C\"]"  ClassName=multi_coupled_C  SchemaVersion=1  noph=3  C=C F
      settings: CopyFcn=simscape.sscblock.internal.componentBlockCallback(gcbh,'COPY')  PreCopyFcn=simscape.sscblock.internal.componentBlockCallback(gcbh,'PRECOPY')  PreDeleteFcn=simscape.sscblock.internal.componentBlockCallback(gcbh,'PREDELETE')  InternalSimscapePortConfiguration="{\"Bottom\":[],\"Left\":[{\"id\":\"p\",\"label\":\"p\",\"type\":\"foundation.electrical.electrical\"}],\"Right\":[{\"id\":\"n\",\"label\":\"n\",\"type\":\"foundation.electrical.electrical\"}],\"Top\":[]}"
      mask Type: Multi-Phase Coupled C
  Mutual RL : SimscapeComponentBlock  SourceFile=multi_coupled_RL  ComponentPath=multi_coupled_RL  ComponentVariants="[\"multi_coupled_RL\"]"  ComponentVariantNames="[\"multi_coupled_RL\"]"  ClassName=multi_coupled_RL  SchemaVersion=1  noph=3  R=R Ohm  L=L H
      settings: CopyFcn=simscape.sscblock.internal.componentBlockCallback(gcbh,'COPY')  PreCopyFcn=simscape.sscblock.internal.componentBlockCallback(gcbh,'PRECOPY')  PreDeleteFcn=simscape.sscblock.internal.componentBlockCallback(gcbh,'PREDELETE')  InternalSimscapePortConfiguration="{\"Bottom\":[],\"Left\":[{\"id\":\"p\",\"label\":\"p\",\"type\":\"foundation.electrical.electrical\"}],\"Right\":[{\"id\":\"n\",\"label\":\"n\",\"type\":\"foundation.electrical.electrical\"}],\"Top\":[]}"
      mask Type: Multi-Phase Coupled RL
  PS-Simulink Converter : nesl_utility/PS-Simulink Converter  PhysicalDomain=network_engine_domain  SubClassName=ps_output  LeftPortType=input  RightPortType=output  PseudoPeriodic=off  Frequencies=[]  VectorFormat=inherit  Unit=inherit  AffineConversion=off
  Simscape Component : SimscapeComponentBlock  SourceFile=multi_current  ComponentPath=multi_current  ComponentVariants="[\"multi_current\"]"  ComponentVariantNames="[\"multi_current\"]"  ClassName=multi_current  SchemaVersion=1  noph=3
      settings: CopyFcn=simscape.sscblock.internal.componentBlockCallback(gcbh,'COPY')  PreCopyFcn=simscape.sscblock.internal.componentBlockCallback(gcbh,'PRECOPY')  PreDeleteFcn=simscape.sscblock.internal.componentBlockCallback(gcbh,'PREDELETE')  InternalSimscapePortConfiguration="{\"Bottom\":[],\"Left\":[{\"id\":\"p\",\"label\":\"+\",\"type\":\"foundation.electrical.electrical\"}],\"Right\":[{\"id\":\"I\",\"label\":\"I\",\"type\":\"output\"},{\"id\":\"n\",\"label\":\"-\",\"type\":\"foundation.electrical.electrical\"}],\"Top\":[]}"
      mask Type: Multi-Phase Current Sensor
  A : PMIOPort  Side=Left
  B : PMIOPort  Port=2  Side=Left
  C : PMIOPort  Port=3  Side=Left
  a : PMIOPort  Port=4  Side=Right
  b : PMIOPort  Port=5  Side=Right
  c : PMIOPort  Port=6  Side=Right
  Imeas : Outport
  wires:
  PS-Simulink Converter/1 -> Imeas/1
  connections:
  c/RConn1 -- Array Connection1/LConn3
  b/RConn1 -- Array Connection1/LConn2
  a/RConn1 -- Array Connection1/LConn1
  C/RConn1 -- Array Connection/LConn3
  B/RConn1 -- Array Connection/LConn2
  A/RConn1 -- Array Connection/LConn1
  Array Connection3/RConn1 -- Mutual C2/RConn1
  PS-Simulink Converter/LConn1 -- Simscape Component/RConn1
  Array Connection/RConn1 -- Simscape Component/LConn1
  Array Connection2/RConn1 -- Mutual C1/RConn1
  Electrical Reference1/LConn1 -- Array Connection3/LConn3 -- Array Connection3/LConn2 -- Array Connection3/LConn1
  Mutual RL/LConn1 -- Simscape Component/RConn2 -- Mutual C1/LConn1
  Mutual C2/LConn1 -- Array Connection1/RConn1 -- Mutual RL/RConn1
  Electrical Reference/LConn1 -- Array Connection2/LConn1 -- Array Connection2/LConn3 -- Array Connection2/LConn2

== system line_choices_snt/T1sscT/OLTC ==
  Electrical Reference : fl_lib/Electrical/Electrical Elements/Electrical Reference
  Electrical Reference1 : fl_lib/Electrical/Electrical Elements/Electrical Reference
  TA : Subsystem
  A : PMIOPort  Tag=PMCPort  Side=Left
  a : PMIOPort  Tag=PMCPort  Port=2  Side=Right
  connections:
  TA/LConn1 -- A/RConn1
  a/RConn1 -- TA/RConn1
  TA/LConn2 -- Electrical Reference/LConn1
  Electrical Reference1/LConn1 -- TA/RConn2

== system line_choices_snt/T1sscT/Pi-Section Line ==
  Electrical Reference : fl_lib/Electrical/Electrical Elements/Electrical Reference
  Electrical Reference1 : fl_lib/Electrical/Electrical Elements/Electrical Reference
  Mutual C1 : SimscapeComponentBlock  SourceFile=multi_coupled_C  ComponentPath=multi_coupled_C  ComponentVariants="[\"multi_coupled_C\"]"  ComponentVariantNames="[\"multi_coupled_C\"]"  ClassName=multi_coupled_C  SchemaVersion=1  noph=1  C=C F
      settings: CopyFcn=simscape.sscblock.internal.componentBlockCallback(gcbh,'COPY')  PreCopyFcn=simscape.sscblock.internal.componentBlockCallback(gcbh,'PRECOPY')  PreDeleteFcn=simscape.sscblock.internal.componentBlockCallback(gcbh,'PREDELETE')  InternalSimscapePortConfiguration="{\"Bottom\":[],\"Left\":[{\"id\":\"p\",\"label\":\"p\",\"type\":\"foundation.electrical.electrical\"}],\"Right\":[{\"id\":\"n\",\"label\":\"n\",\"type\":\"foundation.electrical.electrical\"}],\"Top\":[]}"
      mask Type: Multi-Phase Coupled C
  Mutual C2 : SimscapeComponentBlock  SourceFile=multi_coupled_C  ComponentPath=multi_coupled_C  ComponentVariants="[\"multi_coupled_C\"]"  ComponentVariantNames="[\"multi_coupled_C\"]"  ClassName=multi_coupled_C  SchemaVersion=1  noph=1  C=C F
      settings: CopyFcn=simscape.sscblock.internal.componentBlockCallback(gcbh,'COPY')  PreCopyFcn=simscape.sscblock.internal.componentBlockCallback(gcbh,'PRECOPY')  PreDeleteFcn=simscape.sscblock.internal.componentBlockCallback(gcbh,'PREDELETE')  InternalSimscapePortConfiguration="{\"Bottom\":[],\"Left\":[{\"id\":\"p\",\"label\":\"p\",\"type\":\"foundation.electrical.electrical\"}],\"Right\":[{\"id\":\"n\",\"label\":\"n\",\"type\":\"foundation.electrical.electrical\"}],\"Top\":[]}"
      mask Type: Multi-Phase Coupled C
  Mutual RL : SimscapeComponentBlock  SourceFile=multi_coupled_RL  ComponentPath=multi_coupled_RL  ComponentVariants="[\"multi_coupled_RL\"]"  ComponentVariantNames="[\"multi_coupled_RL\"]"  ClassName=multi_coupled_RL  SchemaVersion=1  noph=1  R=R Ohm  L=L H
      settings: CopyFcn=simscape.sscblock.internal.componentBlockCallback(gcbh,'COPY')  PreCopyFcn=simscape.sscblock.internal.componentBlockCallback(gcbh,'PRECOPY')  PreDeleteFcn=simscape.sscblock.internal.componentBlockCallback(gcbh,'PREDELETE')  InternalSimscapePortConfiguration="{\"Bottom\":[],\"Left\":[{\"id\":\"p\",\"label\":\"p\",\"type\":\"foundation.electrical.electrical\"}],\"Right\":[{\"id\":\"n\",\"label\":\"n\",\"type\":\"foundation.electrical.electrical\"}],\"Top\":[]}"
      mask Type: Multi-Phase Coupled RL
  PS-Simulink Converter : nesl_utility/PS-Simulink Converter  PhysicalDomain=network_engine_domain  SubClassName=ps_output  LeftPortType=input  RightPortType=output  PseudoPeriodic=off  Frequencies=[]  VectorFormat=inherit  Unit=inherit  AffineConversion=off
  Simscape Component : SimscapeComponentBlock  SourceFile=multi_current  ComponentPath=multi_current  ComponentVariants="[\"multi_current\"]"  ComponentVariantNames="[\"multi_current\"]"  ClassName=multi_current  SchemaVersion=1  noph=1
      settings: CopyFcn=simscape.sscblock.internal.componentBlockCallback(gcbh,'COPY')  PreCopyFcn=simscape.sscblock.internal.componentBlockCallback(gcbh,'PRECOPY')  PreDeleteFcn=simscape.sscblock.internal.componentBlockCallback(gcbh,'PREDELETE')  InternalSimscapePortConfiguration="{\"Bottom\":[],\"Left\":[{\"id\":\"p\",\"label\":\"+\",\"type\":\"foundation.electrical.electrical\"}],\"Right\":[{\"id\":\"I\",\"label\":\"I\",\"type\":\"output\"},{\"id\":\"n\",\"label\":\"-\",\"type\":\"foundation.electrical.electrical\"}],\"Top\":[]}"
      mask Type: Multi-Phase Current Sensor
  A : PMIOPort  Side=Left
  a : PMIOPort  Port=2  Side=Right
  Imeas : Outport
  wires:
  PS-Simulink Converter/1 -> Imeas/1
  connections:
  Mutual RL/LConn1 -- Simscape Component/RConn2 -- Mutual C1/LConn1
  Mutual RL/RConn1 -- a/RConn1 -- Mutual C2/LConn1
  Mutual C1/RConn1 -- Electrical Reference/LConn1
  Mutual C2/RConn1 -- Electrical Reference1/LConn1
  Simscape Component/LConn1 -- A/RConn1
  PS-Simulink Converter/LConn1 -- Simscape Component/RConn1

== system line_choices_snt/T1sscTf/OLTC ==
  Electrical Reference : fl_lib/Electrical/Electrical Elements/Electrical Reference
  Electrical Reference1 : fl_lib/Electrical/Electrical Elements/Electrical Reference
  TA : Subsystem
  A : PMIOPort  Tag=PMCPort  Side=Left
  a : PMIOPort  Tag=PMCPort  Port=2  Side=Right
  connections:
  Electrical Reference1/LConn1 -- TA/RConn2
  TA/LConn2 -- Electrical Reference/LConn1
  a/RConn1 -- TA/RConn1
  TA/LConn1 -- A/RConn1

== system line_choices_snt/T1sscTf/Pi-Section Line ==
  Electrical Reference : fl_lib/Electrical/Electrical Elements/Electrical Reference
  Electrical Reference1 : fl_lib/Electrical/Electrical Elements/Electrical Reference
  Mutual C1 : SimscapeComponentBlock  SourceFile=multi_coupled_C  ComponentPath=multi_coupled_C  ComponentVariants="[\"multi_coupled_C\"]"  ComponentVariantNames="[\"multi_coupled_C\"]"  ClassName=multi_coupled_C  SchemaVersion=1  noph=1  C=C F
      settings: CopyFcn=simscape.sscblock.internal.componentBlockCallback(gcbh,'COPY')  PreCopyFcn=simscape.sscblock.internal.componentBlockCallback(gcbh,'PRECOPY')  PreDeleteFcn=simscape.sscblock.internal.componentBlockCallback(gcbh,'PREDELETE')  InternalSimscapePortConfiguration="{\"Bottom\":[],\"Left\":[{\"id\":\"p\",\"label\":\"p\",\"type\":\"foundation.electrical.electrical\"}],\"Right\":[{\"id\":\"n\",\"label\":\"n\",\"type\":\"foundation.electrical.electrical\"}],\"Top\":[]}"
      mask Type: Multi-Phase Coupled C
  Mutual C2 : SimscapeComponentBlock  SourceFile=multi_coupled_C  ComponentPath=multi_coupled_C  ComponentVariants="[\"multi_coupled_C\"]"  ComponentVariantNames="[\"multi_coupled_C\"]"  ClassName=multi_coupled_C  SchemaVersion=1  noph=1  C=C F
      settings: CopyFcn=simscape.sscblock.internal.componentBlockCallback(gcbh,'COPY')  PreCopyFcn=simscape.sscblock.internal.componentBlockCallback(gcbh,'PRECOPY')  PreDeleteFcn=simscape.sscblock.internal.componentBlockCallback(gcbh,'PREDELETE')  InternalSimscapePortConfiguration="{\"Bottom\":[],\"Left\":[{\"id\":\"p\",\"label\":\"p\",\"type\":\"foundation.electrical.electrical\"}],\"Right\":[{\"id\":\"n\",\"label\":\"n\",\"type\":\"foundation.electrical.electrical\"}],\"Top\":[]}"
      mask Type: Multi-Phase Coupled C
  Mutual RL : SimscapeComponentBlock  SourceFile=multi_coupled_RL  ComponentPath=multi_coupled_RL  ComponentVariants="[\"multi_coupled_RL\"]"  ComponentVariantNames="[\"multi_coupled_RL\"]"  ClassName=multi_coupled_RL  SchemaVersion=1  noph=1  R=R Ohm  L=L H
      settings: CopyFcn=simscape.sscblock.internal.componentBlockCallback(gcbh,'COPY')  PreCopyFcn=simscape.sscblock.internal.componentBlockCallback(gcbh,'PRECOPY')  PreDeleteFcn=simscape.sscblock.internal.componentBlockCallback(gcbh,'PREDELETE')  InternalSimscapePortConfiguration="{\"Bottom\":[],\"Left\":[{\"id\":\"p\",\"label\":\"p\",\"type\":\"foundation.electrical.electrical\"}],\"Right\":[{\"id\":\"n\",\"label\":\"n\",\"type\":\"foundation.electrical.electrical\"}],\"Top\":[]}"
      mask Type: Multi-Phase Coupled RL
  PS-Simulink Converter : nesl_utility/PS-Simulink Converter  PhysicalDomain=network_engine_domain  SubClassName=ps_output  LeftPortType=input  RightPortType=output  PseudoPeriodic=off  Frequencies=[]  VectorFormat=inherit  Unit=inherit  AffineConversion=off
  Simscape Component : SimscapeComponentBlock  SourceFile=multi_current  ComponentPath=multi_current  ComponentVariants="[\"multi_current\"]"  ComponentVariantNames="[\"multi_current\"]"  ClassName=multi_current  SchemaVersion=1  noph=1
      settings: CopyFcn=simscape.sscblock.internal.componentBlockCallback(gcbh,'COPY')  PreCopyFcn=simscape.sscblock.internal.componentBlockCallback(gcbh,'PRECOPY')  PreDeleteFcn=simscape.sscblock.internal.componentBlockCallback(gcbh,'PREDELETE')  InternalSimscapePortConfiguration="{\"Bottom\":[],\"Left\":[{\"id\":\"p\",\"label\":\"+\",\"type\":\"foundation.electrical.electrical\"}],\"Right\":[{\"id\":\"I\",\"label\":\"I\",\"type\":\"output\"},{\"id\":\"n\",\"label\":\"-\",\"type\":\"foundation.electrical.electrical\"}],\"Top\":[]}"
      mask Type: Multi-Phase Current Sensor
  A : PMIOPort  Side=Left
  a : PMIOPort  Port=2  Side=Right
  Imeas : Outport
  wires:
  PS-Simulink Converter/1 -> Imeas/1
  connections:
  PS-Simulink Converter/LConn1 -- Simscape Component/RConn1
  Simscape Component/LConn1 -- A/RConn1
  Mutual C2/RConn1 -- Electrical Reference1/LConn1
  Mutual C1/RConn1 -- Electrical Reference/LConn1
  Mutual C2/LConn1 -- a/RConn1 -- Mutual RL/RConn1
  Mutual C1/LConn1 -- Simscape Component/RConn2 -- Mutual RL/LConn1
